simulink model "Train10"  (R2020a)
settings: Solver=VariableStepAuto  StartTime=0.0  StopTime=10.0  RelTol=1e-3
undefined symbols (not defined in the file): c, k, M_1, M_10, M_2, M_3, M_4, M_5, M_6, M_7, M_8, M_9, X0_10, X0_2, X0_3, X0_4, X0_5, X0_6, X0_7, X0_8, X0_9
settings Model: OrderedModelArguments=off  Creator=zhenya  LastModifiedBy=zhenya
settings DebuggingCC: ArithmeticOperatorsInVariantConditions=warning
settings SFSimCC: CustomCodeUndefinedFunction=UseInterfaceOnly

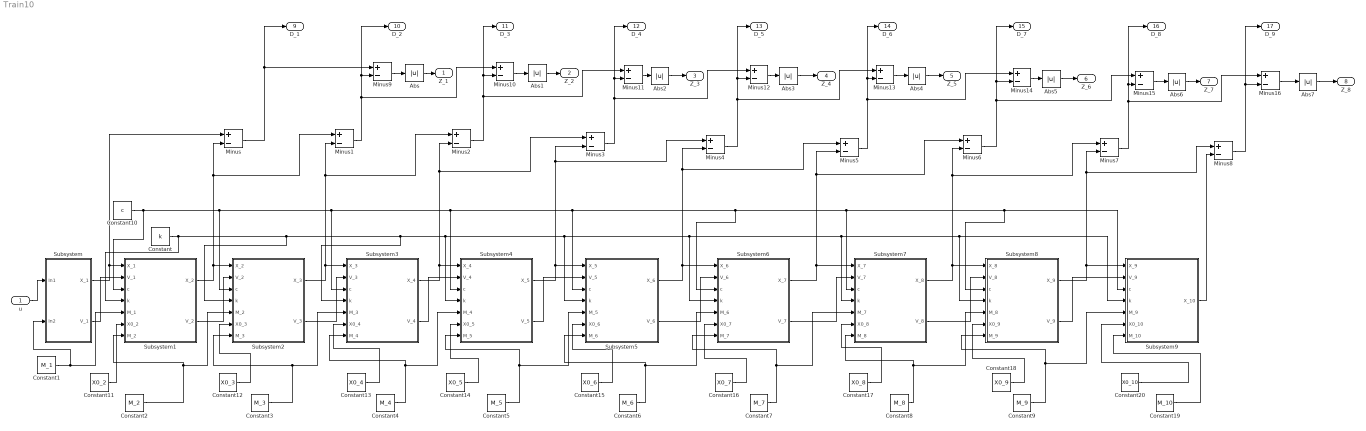
== system Train10 ==
  u : Inport
  Abs{,1..7} (8 alike) : Abs
  Constant : Constant  Value=k
  Constant1 : Constant  Value=M_1
  Constant10 : Constant  Value=c
  Constant11 : Constant  Value=X0_2
  Constant12 : Constant  Value=X0_3
  Constant13 : Constant  Value=X0_4
  Constant14 : Constant  Value=X0_5
  Constant15 : Constant  Value=X0_6
  Constant16 : Constant  Value=X0_7
  Constant17 : Constant  Value=X0_8
  Constant18 : Constant  Value=X0_9
  Constant19 : Constant  Value=M_10
  Constant2 : Constant  Value=M_2
  Constant20 : Constant  Value=X0_10
  Constant3 : Constant  Value=M_3
  Constant4 : Constant  Value=M_4
  Constant5 : Constant  Value=M_5
  Constant6 : Constant  Value=M_6
  Constant7 : Constant  Value=M_7
  Constant8 : Constant  Value=M_8
  Constant9 : Constant  Value=M_9
  Minus{,1..16} (17 alike) : Sum  Inputs=+-
  Subsystem : Subsystem
  Subsystem1 : Subsystem
  Subsystem2 : Subsystem
  Subsystem3 : Subsystem
  Subsystem4 : Subsystem
  Subsystem5 : Subsystem
  Subsystem6 : Subsystem
  Subsystem7 : Subsystem
  Subsystem8 : Subsystem
  Subsystem9 : Subsystem
  Z_1 : Outport
  Z_2 : Outport  Port=2
  Z_3 : Outport  Port=3
  Z_4 : Outport  Port=4
  Z_5 : Outport  Port=5
  Z_6 : Outport  Port=6
  Z_7 : Outport  Port=7
  Z_8 : Outport  Port=8
  D_1 : Outport  Port=9
  D_2 : Outport  Port=10
  D_3 : Outport  Port=11
  D_4 : Outport  Port=12
  D_5 : Outport  Port=13
  D_6 : Outport  Port=14
  D_7 : Outport  Port=15
  D_8 : Outport  Port=16
  D_9 : Outport  Port=17
  wires:
  u/1 -> Subsystem/1(In1)
  Constant/1 -> Subsystem9/4(k), Subsystem8/4(k), Subsystem7/4(k), Subsystem6/4(k), Subsystem5/4(k), Subsystem4/4(k), Subsystem3/4(k), Subsystem2/4(k), Subsystem1/4(k)
  Constant2/1 -> Subsystem2/5(M_2), Subsystem1/7(M_2)
  Subsystem/2(V_1) -> Subsystem1/2(V_1)
  Constant10/1 -> Subsystem9/3(c), Subsystem8/3(c), Subsystem7/3(c), Subsystem6/3(c), Subsystem5/3(c), Subsystem4/3(c), Subsystem3/3(c), Subsystem2/3(c), Subsystem1/3(c)
  Constant1/1 -> Subsystem1/5(M_1), Subsystem/2(In2)
  Subsystem1/1(X_2) -> Minus1/1, Minus/2, Subsystem2/1(X_2)
  Subsystem1/2(V_2) -> Subsystem2/2(V_2)
  Constant3/1 -> Subsystem3/5(M_3), Subsystem2/7(M_3)
  Subsystem2/1(X_3) -> Minus2/1, Minus1/2, Subsystem3/1(X_3)
  Subsystem2/2(V_3) -> Subsystem3/2(V_3)
  Constant4/1 -> Subsystem4/5(M_4), Subsystem3/7(M_4)
  Subsystem3/2(V_4) -> Subsystem4/2(V_4)
  Subsystem3/1(X_4) -> Minus3/1, Minus2/2, Subsystem4/1(X_4)
  Constant5/1 -> Subsystem5/5(M_5), Subsystem4/7(M_5)
  Subsystem4/1(X_5) -> Minus4/1, Minus3/2, Subsystem5/1(X_5)
  Subsystem4/2(V_5) -> Subsystem5/2(V_5)
  Constant6/1 -> Subsystem6/5(M_6), Subsystem5/7(M_6)
  Subsystem5/1(X_6) -> Minus5/1, Minus4/2, Subsystem6/1(X_6)
  Subsystem5/2(V_6) -> Subsystem6/2(V_6)
  Constant7/1 -> Subsystem7/5(M_7), Subsystem6/7(M_7)
  Subsystem6/1(X_7) -> Minus6/1, Minus5/2, Subsystem7/1(X_7)
  Subsystem6/2(V_7) -> Subsystem7/2(V_7)
  Constant8/1 -> Subsystem8/5(M_8), Subsystem7/7(M_8)
  Subsystem7/1(X_8) -> Minus7/1, Minus6/2, Subsystem8/1(X_8)
  Subsystem7/2(V_8) -> Subsystem8/2(V_8)
  Constant9/1 -> Subsystem9/5(M_9), Subsystem8/7(M_9)
  Subsystem8/1(X_9) -> Subsystem9/1(X_9), Minus8/1, Minus7/2
  Subsystem/1(X_1) -> Minus/1, Subsystem1/1(X_1)
  Minus/1 -> D_1/1, Minus9/1
  Minus1/1 -> Minus10/1, D_2/1, Minus9/2
  Minus2/1 -> Minus11/1, D_3/1, Minus10/2
  Minus3/1 -> Minus12/1, D_4/1, Minus11/2
  Minus4/1 -> Minus13/1, D_5/1, Minus12/2
  Minus5/1 -> Minus14/1, D_6/1, Minus13/2
  Minus6/1 -> Minus15/1, D_7/1, Minus14/2
  Minus7/1 -> Minus16/1, D_8/1, Minus15/2
  Constant11/1 -> Subsystem1/6(X0_2)
  Constant12/1 -> Subsystem2/6(X0_3)
  Constant13/1 -> Subsystem3/6(X0_4)
  Constant14/1 -> Subsystem4/6(X0_5)
  Constant15/1 -> Subsystem5/6(X0_6)
  Constant16/1 -> Subsystem6/6(X0_7)
  Constant17/1 -> Subsystem7/6(X0_8)
  Constant18/1 -> Subsystem8/6(X0_9)
  Subsystem8/2(V_9) -> Subsystem9/2(V_9)
  Constant19/1 -> Subsystem9/7(M_10)
  Constant20/1 -> Subsystem9/6(X0_10)
  Subsystem9/1(X_10) -> Minus8/2
  Minus8/1 -> D_9/1, Minus16/2
  Minus9/1 -> Abs/1
  Abs/1 -> Z_1/1
  Minus10/1 -> Abs1/1
  Abs1/1 -> Z_2/1
  Minus11/1 -> Abs2/1
  Abs2/1 -> Z_3/1
  Minus12/1 -> Abs3/1
  Abs3/1 -> Z_4/1
  Minus13/1 -> Abs4/1
  Abs4/1 -> Z_5/1
  Minus14/1 -> Abs5/1
  Abs5/1 -> Z_6/1
  Minus15/1 -> Abs6/1
  Abs6/1 -> Z_7/1
  Minus16/1 -> Abs7/1
  Abs7/1 -> Z_8/1

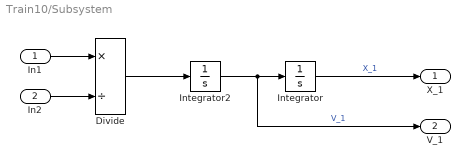
== system Train10/Subsystem ==
  In1 : Inport
  In2 : Inport  Port=2
  Divide : Product  Inputs=*/
  Integrator : Integrator
  Integrator2 : Integrator
  X_1 : Outport
  V_1 : Outport  Port=2
  wires:
  Integrator/1 -> X_1/1  "X_1"
  Integrator2/1 -> V_1/1, Integrator/1  "V_1"
  In1/1 -> Divide/1
  In2/1 -> Divide/2
  Divide/1 -> Integrator2/1

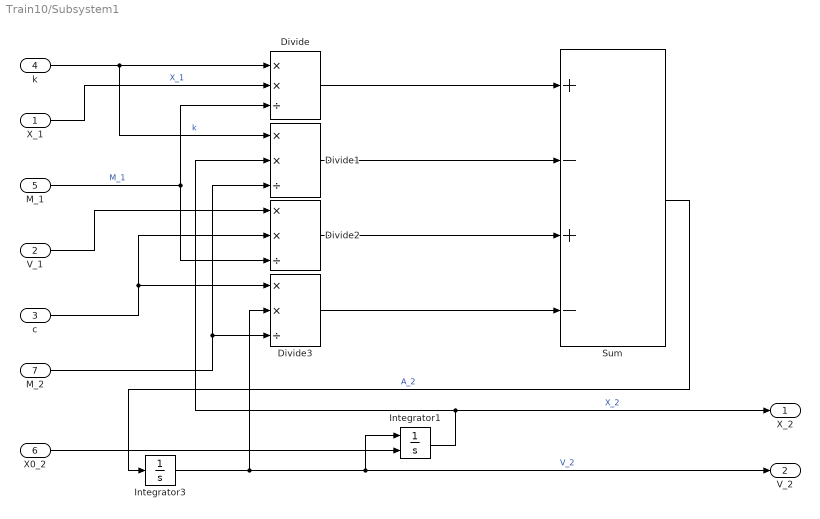
== system Train10/Subsystem1 ==
  X_1 : Inport
  V_1 : Inport  Port=2
  c : Inport  Port=3
  k : Inport  Port=4
  M_1 : Inport  Port=5
  X0_2 : Inport  Port=6
  M_2 : Inport  Port=7
  Divide{,1..3} (4 alike) : Product  Inputs=**/
  Integrator1 : Integrator  InitialConditionSource=external
  Integrator3 : Integrator
  Sum : Sum  Inputs=+-+-
  X_2 : Outport
  V_2 : Outport  Port=2
  wires:
  Divide2/1 -> Sum/3
  X_1/1 -> Divide/2  "X_1"
  Integrator3/1 -> Integrator1/1, V_2/1, Divide3/2  "V_2"
  Divide1/1 -> Sum/2
  V_1/1 -> Divide2/1
  Divide3/1 -> Sum/4
  Integrator1/1 -> Divide1/2, X_2/1  "X_2"
  Sum/1 -> Integrator3/1  "A_2"
  k/1 -> Divide1/1, Divide/1  "k"
  M_1/1 -> Divide2/3, Divide/3  "M_1"
  Divide/1 -> Sum/1
  M_2/1 -> Divide3/3, Divide1/3
  c/1 -> Divide2/2, Divide3/1
  X0_2/1 -> Integrator1/2

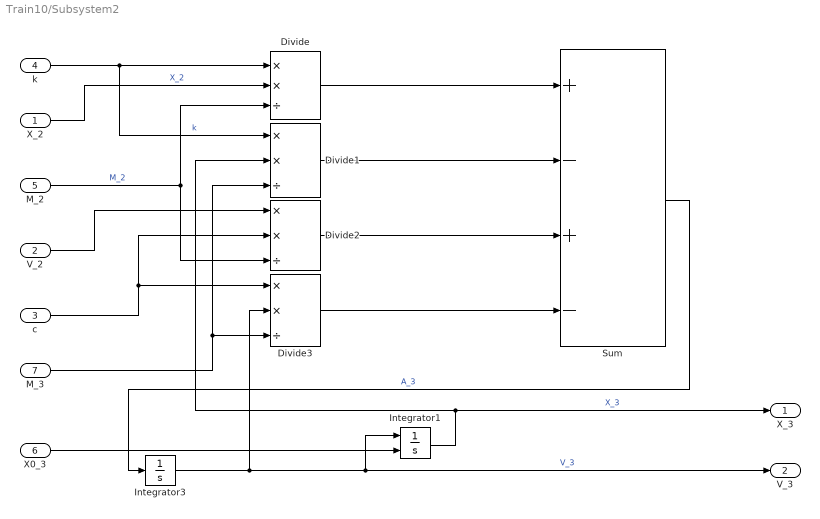
== system Train10/Subsystem2 ==
  X_2 : Inport
  V_2 : Inport  Port=2
  c : Inport  Port=3
  k : Inport  Port=4
  M_2 : Inport  Port=5
  X0_3 : Inport  Port=6
  M_3 : Inport  Port=7
  Divide{,1..3} (4 alike) : Product  Inputs=**/
  Integrator1 : Integrator  InitialConditionSource=external  InitialCondition=-28
  Integrator3 : Integrator
  Sum : Sum  Inputs=+-+-
  X_3 : Outport
  V_3 : Outport  Port=2
  wires:
  Divide2/1 -> Sum/3
  X_2/1 -> Divide/2  "X_2"
  Integrator3/1 -> Integrator1/1, V_3/1, Divide3/2  "V_3"
  Divide1/1 -> Sum/2
  V_2/1 -> Divide2/1
  Divide3/1 -> Sum/4
  Integrator1/1 -> Divide1/2, X_3/1  "X_3"
  Sum/1 -> Integrator3/1  "A_3"
  k/1 -> Divide1/1, Divide/1  "k"
  M_2/1 -> Divide2/3, Divide/3  "M_2"
  Divide/1 -> Sum/1
  M_3/1 -> Divide3/3, Divide1/3
  c/1 -> Divide2/2, Divide3/1
  X0_3/1 -> Integrator1/2

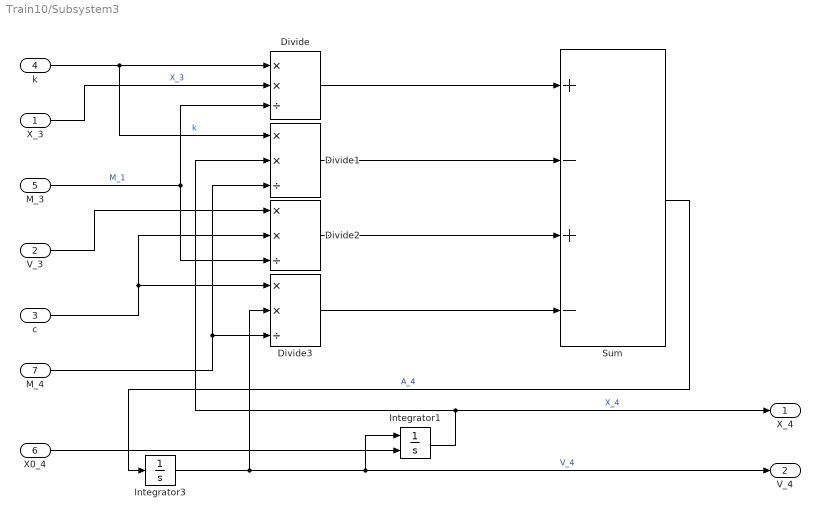
== system Train10/Subsystem3 ==
  X_3 : Inport
  V_3 : Inport  Port=2
  c : Inport  Port=3
  k : Inport  Port=4
  M_3 : Inport  Port=5
  X0_4 : Inport  Port=6
  M_4 : Inport  Port=7
  Divide{,1..3} (4 alike) : Product  Inputs=**/
  Integrator1 : Integrator  InitialConditionSource=external  InitialCondition=-40.5
  Integrator3 : Integrator
  Sum : Sum  Inputs=+-+-
  X_4 : Outport
  V_4 : Outport  Port=2
  wires:
  Divide2/1 -> Sum/3
  X_3/1 -> Divide/2  "X_3"
  Integrator3/1 -> Integrator1/1, V_4/1, Divide3/2  "V_4"
  Divide1/1 -> Sum/2
  V_3/1 -> Divide2/1
  Divide3/1 -> Sum/4
  Integrator1/1 -> Divide1/2, X_4/1  "X_4"
  Sum/1 -> Integrator3/1  "A_4"
  k/1 -> Divide1/1, Divide/1  "k"
  M_3/1 -> Divide2/3, Divide/3  "M_1"
  Divide/1 -> Sum/1
  M_4/1 -> Divide3/3, Divide1/3
  c/1 -> Divide2/2, Divide3/1
  X0_4/1 -> Integrator1/2

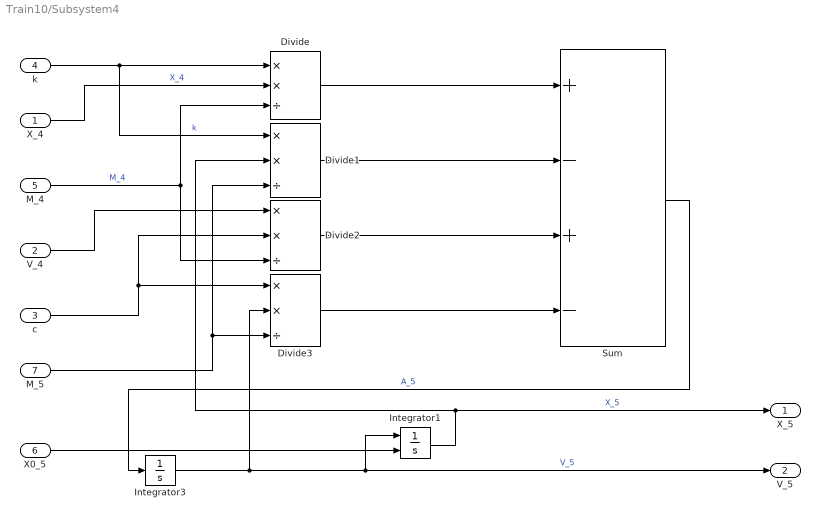
== system Train10/Subsystem4 ==
  X_4 : Inport
  V_4 : Inport  Port=2
  c : Inport  Port=3
  k : Inport  Port=4
  M_4 : Inport  Port=5
  X0_5 : Inport  Port=6
  M_5 : Inport  Port=7
  Divide{,1..3} (4 alike) : Product  Inputs=**/
  Integrator1 : Integrator  InitialConditionSource=external  InitialCondition=-52
  Integrator3 : Integrator
  Sum : Sum  Inputs=+-+-
  X_5 : Outport
  V_5 : Outport  Port=2
  wires:
  Divide2/1 -> Sum/3
  X_4/1 -> Divide/2  "X_4"
  Integrator3/1 -> Integrator1/1, V_5/1, Divide3/2  "V_5"
  Divide1/1 -> Sum/2
  V_4/1 -> Divide2/1
  Divide3/1 -> Sum/4
  Integrator1/1 -> Divide1/2, X_5/1  "X_5"
  Sum/1 -> Integrator3/1  "A_5"
  k/1 -> Divide1/1, Divide/1  "k"
  M_4/1 -> Divide2/3, Divide/3  "M_4"
  Divide/1 -> Sum/1
  M_5/1 -> Divide3/3, Divide1/3
  c/1 -> Divide2/2, Divide3/1
  X0_5/1 -> Integrator1/2

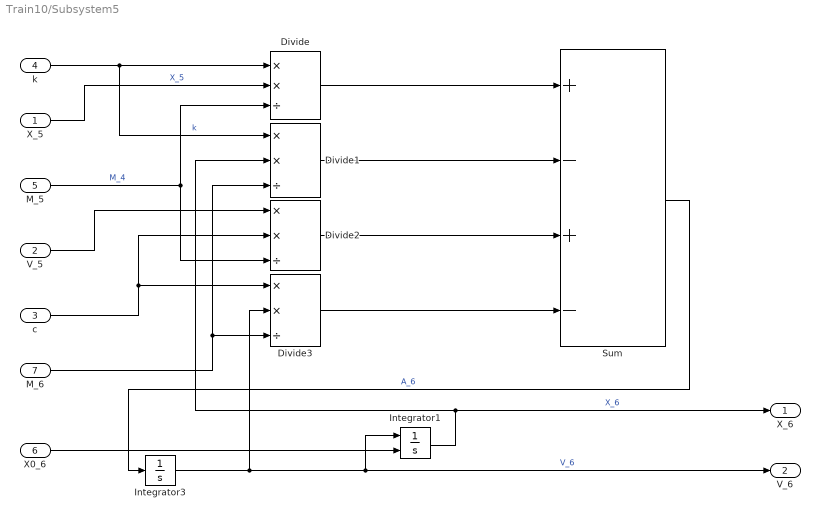
== system Train10/Subsystem5 ==
  X_5 : Inport
  V_5 : Inport  Port=2
  c : Inport  Port=3
  k : Inport  Port=4
  M_5 : Inport  Port=5
  X0_6 : Inport  Port=6
  M_6 : Inport  Port=7
  Divide{,1..3} (4 alike) : Product  Inputs=**/
  Integrator1 : Integrator  InitialConditionSource=external  InitialCondition=-62.5
  Integrator3 : Integrator
  Sum : Sum  Inputs=+-+-
  X_6 : Outport
  V_6 : Outport  Port=2
  wires:
  Divide2/1 -> Sum/3
  X_5/1 -> Divide/2  "X_5"
  Integrator3/1 -> Integrator1/1, V_6/1, Divide3/2  "V_6"
  Divide1/1 -> Sum/2
  V_5/1 -> Divide2/1
  Divide3/1 -> Sum/4
  Integrator1/1 -> Divide1/2, X_6/1  "X_6"
  Sum/1 -> Integrator3/1  "A_6"
  k/1 -> Divide1/1, Divide/1  "k"
  M_5/1 -> Divide2/3, Divide/3  "M_4"
  Divide/1 -> Sum/1
  M_6/1 -> Divide3/3, Divide1/3
  c/1 -> Divide2/2, Divide3/1
  X0_6/1 -> Integrator1/2

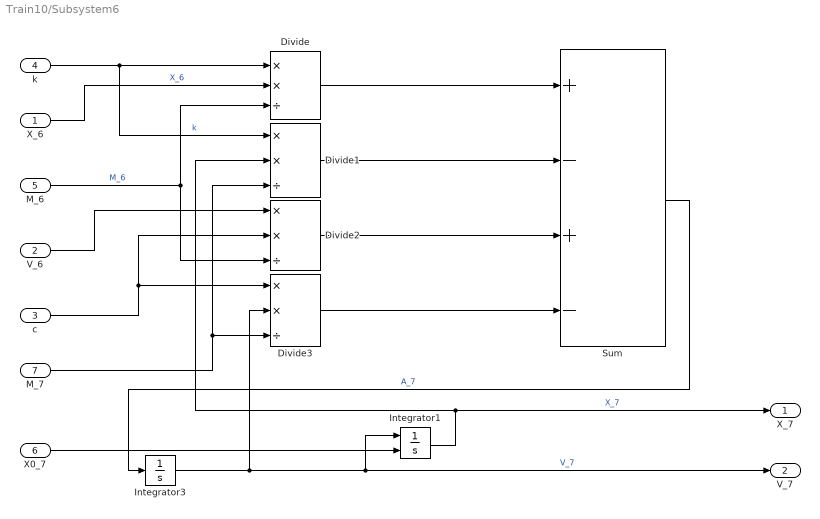
== system Train10/Subsystem6 ==
  X_6 : Inport
  V_6 : Inport  Port=2
  c : Inport  Port=3
  k : Inport  Port=4
  M_6 : Inport  Port=5
  X0_7 : Inport  Port=6
  M_7 : Inport  Port=7
  Divide{,1..3} (4 alike) : Product  Inputs=**/
  Integrator1 : Integrator  InitialConditionSource=external  InitialCondition=-72
  Integrator3 : Integrator
  Sum : Sum  Inputs=+-+-
  X_7 : Outport
  V_7 : Outport  Port=2
  wires:
  Divide2/1 -> Sum/3
  X_6/1 -> Divide/2  "X_6"
  Integrator3/1 -> Integrator1/1, V_7/1, Divide3/2  "V_7"
  Divide1/1 -> Sum/2
  V_6/1 -> Divide2/1
  Divide3/1 -> Sum/4
  Integrator1/1 -> Divide1/2, X_7/1  "X_7"
  Sum/1 -> Integrator3/1  "A_7"
  k/1 -> Divide1/1, Divide/1  "k"
  M_6/1 -> Divide2/3, Divide/3  "M_6"
  Divide/1 -> Sum/1
  M_7/1 -> Divide3/3, Divide1/3
  c/1 -> Divide2/2, Divide3/1
  X0_7/1 -> Integrator1/2

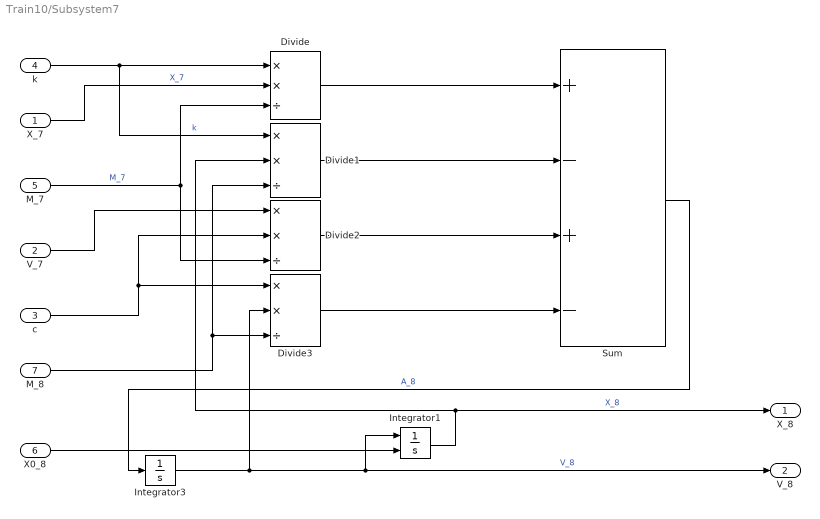
== system Train10/Subsystem7 ==
  X_7 : Inport
  V_7 : Inport  Port=2
  c : Inport  Port=3
  k : Inport  Port=4
  M_7 : Inport  Port=5
  X0_8 : Inport  Port=6
  M_8 : Inport  Port=7
  Divide{,1..3} (4 alike) : Product  Inputs=**/
  Integrator1 : Integrator  InitialConditionSource=external  InitialCondition=-80.5
  Integrator3 : Integrator
  Sum : Sum  Inputs=+-+-
  X_8 : Outport
  V_8 : Outport  Port=2
  wires:
  Divide2/1 -> Sum/3
  X_7/1 -> Divide/2  "X_7"
  Integrator3/1 -> Integrator1/1, V_8/1, Divide3/2  "V_8"
  Divide1/1 -> Sum/2
  V_7/1 -> Divide2/1
  Divide3/1 -> Sum/4
  Integrator1/1 -> Divide1/2, X_8/1  "X_8"
  Sum/1 -> Integrator3/1  "A_8"
  k/1 -> Divide1/1, Divide/1  "k"
  M_7/1 -> Divide2/3, Divide/3  "M_7"
  Divide/1 -> Sum/1
  M_8/1 -> Divide3/3, Divide1/3
  c/1 -> Divide2/2, Divide3/1
  X0_8/1 -> Integrator1/2

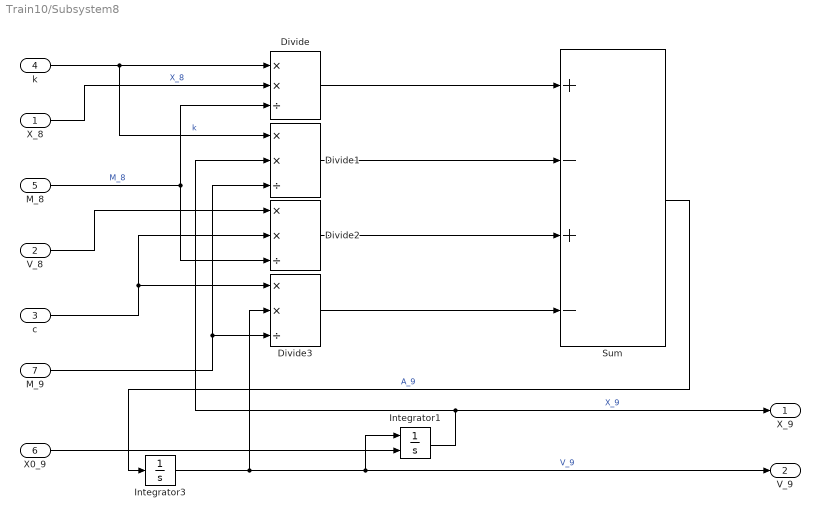
== system Train10/Subsystem8 ==
  X_8 : Inport
  V_8 : Inport  Port=2
  c : Inport  Port=3
  k : Inport  Port=4
  M_8 : Inport  Port=5
  X0_9 : Inport  Port=6
  M_9 : Inport  Port=7
  Divide{,1..3} (4 alike) : Product  Inputs=**/
  Integrator1 : Integrator  InitialConditionSource=external  InitialCondition=-88
  Integrator3 : Integrator
  Sum : Sum  Inputs=+-+-
  X_9 : Outport
  V_9 : Outport  Port=2
  wires:
  Divide2/1 -> Sum/3
  X_8/1 -> Divide/2  "X_8"
  Integrator3/1 -> V_9/1, Integrator1/1, Divide3/2  "V_9"
  Divide1/1 -> Sum/2
  V_8/1 -> Divide2/1
  Divide3/1 -> Sum/4
  Integrator1/1 -> Divide1/2, X_9/1  "X_9"
  Sum/1 -> Integrator3/1  "A_9"
  k/1 -> Divide1/1, Divide/1  "k"
  M_8/1 -> Divide2/3, Divide/3  "M_8"
  Divide/1 -> Sum/1
  M_9/1 -> Divide3/3, Divide1/3
  c/1 -> Divide2/2, Divide3/1
  X0_9/1 -> Integrator1/2

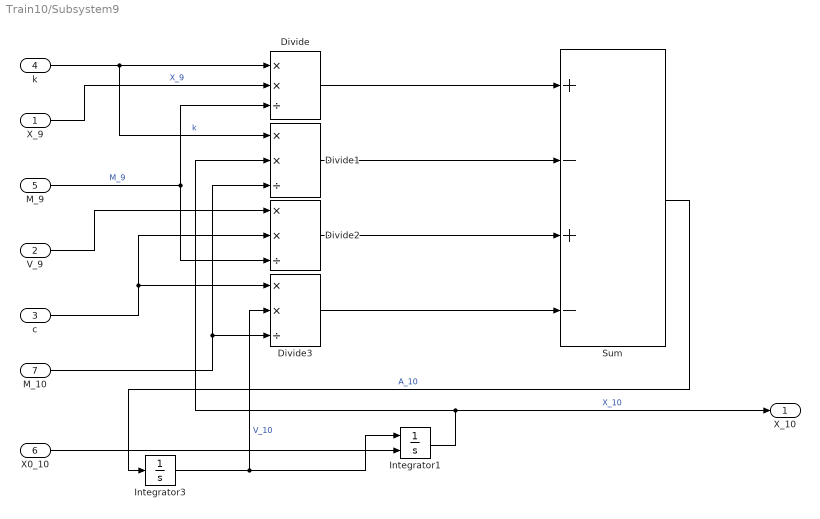
== system Train10/Subsystem9 ==
  X_9 : Inport
  V_9 : Inport  Port=2
  c : Inport  Port=3
  k : Inport  Port=4
  M_9 : Inport  Port=5
  X0_10 : Inport  Port=6
  M_10 : Inport  Port=7
  Divide{,1..3} (4 alike) : Product  Inputs=**/
  Integrator1 : Integrator  InitialConditionSource=external  InitialCondition=-88
  Integrator3 : Integrator
  Sum : Sum  Inputs=+-+-
  X_10 : Outport
  wires:
  Divide2/1 -> Sum/3
  X_9/1 -> Divide/2  "X_9"
  Integrator3/1 -> Integrator1/1, Divide3/2  "V_10"
  Divide1/1 -> Sum/2
  V_9/1 -> Divide2/1
  Divide3/1 -> Sum/4
  Integrator1/1 -> Divide1/2, X_10/1  "X_10"
  Sum/1 -> Integrator3/1  "A_10"
  k/1 -> Divide1/1, Divide/1  "k"
  M_9/1 -> Divide2/3, Divide/3  "M_9"
  Divide/1 -> Sum/1
  M_10/1 -> Divide3/3, Divide1/3
  c/1 -> Divide2/2, Divide3/1
  X0_10/1 -> Integrator1/2
